simulink model "withaudioip"  (R2016a)
settings: Solver=ode45  StartTime=0.0  StopTime=inf  RelTol=1e-3
libraries: audiosources x1, dspadpt3 x1, dspsnks4 x1
settings Model: Creator=richanetto  LastModifiedBy=richanetto
settings SolverCC: AlgebraicLoopSolver=LineSearch
settings DataIOCC: LimitDataPoints=on
settings DebuggingCC: AlgebraicLoopMsg=none
settings HardwareCC: ProdWordSize=32  ProdHWDeviceType=Specified
settings ModelReferenceCC: PropagateSignalLabelsOutOfModel=off
settings GRTTargetCC: GeneratePreprocessorConditionals=Use local settings

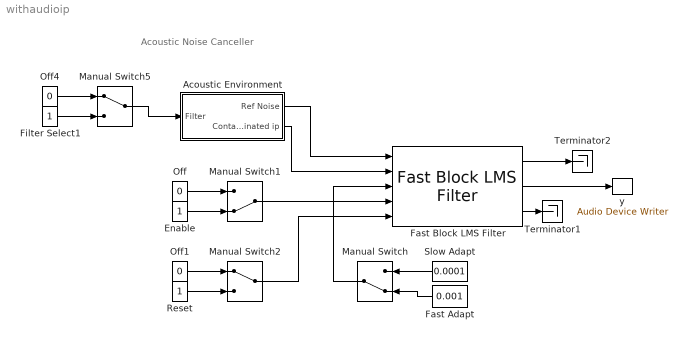
== system withaudioip ==
  note: Acoustic Noise Canceller
  Acoustic Environment : Subsystem
  Enable : Constant  OutDataTypeStr=boolean
  Fast Adapt : Constant  Value=0.001  OutDataTypeStr=Inherit: Inherit via back propagation
  Fast Block LMS Filter : dspadpt3/Fast Block LMS Filter  algo=Fast Block LMS  L=48  N=16  stepflag=Input port  mu=0.008  leakage=1.0  addnparflag=on  ic=0  Adapt=on  resetflag=Non-zero sample  weights=on
  Filter Select1 : Constant  OutDataTypeStr=boolean
  Manual Switch : ManualSwitch  CurrentSetting=0
  Manual Switch1 : ManualSwitch  CurrentSetting=0
  Manual Switch2 : ManualSwitch
  Manual Switch5 : ManualSwitch
  Off : Constant  Value=0  OutDataTypeStr=boolean
  Off1 : Constant  Value=0  OutDataTypeStr=boolean
  Off4 : Constant  Value=0  OutDataTypeStr=boolean
  Reset : Constant  OutDataTypeStr=boolean
  Slow Adapt : Constant  Value=0.0001  OutDataTypeStr=Inherit: Inherit via back propagation
  Terminator1 : Terminator
  Terminator2 : Terminator
  y : dspsnks4/Audio Device Writer  Driver=CoreAudio  Device=Default  InheritSampleRate=on  SampleRate=44100  BitDepth=16-bit integer  BufferSize=4096  NumBuffers=10  DefaultOutputChannelMapping=on  OutputChannelMapping=1:2  OutputNumUnderrunSamples=off  DriverIdx=5  DeviceWarnFlag=''
  wires:
  Slow Adapt/1 -> Manual Switch/1
  Fast Adapt/1 -> Manual Switch/2
  Manual Switch/1 -> Fast Block LMS Filter/3
  Fast Block LMS Filter/3 -> Terminator1/1
  Off/1 -> Manual Switch1/1
  Enable/1 -> Manual Switch1/2
  Off1/1 -> Manual Switch2/1
  Reset/1 -> Manual Switch2/2
  Manual Switch2/1 -> Fast Block LMS Filter/5
  Manual Switch1/1 -> Fast Block LMS Filter/4
  Off4/1 -> Manual Switch5/1
  Filter Select1/1 -> Manual Switch5/2
  Manual Switch5/1 -> Acoustic Environment/1(Filter)
  Acoustic Environment/1(Ref Noise) -> Fast Block LMS Filter/1
  Acoustic Environment/2(Contaminated ip) -> Fast Block LMS Filter/2
  Fast Block LMS Filter/2 -> y/1
  Fast Block LMS Filter/1 -> Terminator2/1

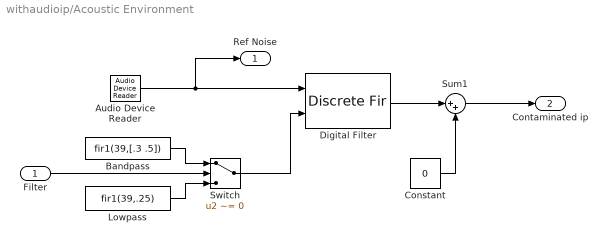
== system withaudioip/Acoustic Environment ==
  Filter : Inport
  Audio Device Reader : audiosources/Audio Device Reader  Driver=CoreAudio  Device=Built-in Microph  SampleRate=44100  NumChannels=1  SamplesPerFrame=1024  BitDepth=16-bit integer  NumBuffers=10  DefaultInputChannelMapping=on  InputChannelMapping=1:2  OutputNumOverrunSamples=off  OutputDataType=double  DriverIdx=5  DeviceWarnFlag=''
  Bandpass : Constant  Value=fir1(39,[.3 .5])  OutDataTypeStr=Inherit: Inherit via back propagation
  Constant : Constant  Value=0
  Digital Filter : DiscreteFir  CoefSource=Input port  Coefficients=[1 2]  InputProcessing=Columns as channels (frame based)  AccumDataTypeStr=Inherit: Same as product output  OutDataTypeStr=Inherit: Same as input
      settings: InputPortMap=u0,u1
  Lowpass : Constant  Value=fir1(39,.25)  OutDataTypeStr=Inherit: Inherit via back propagation
  Sum1 : Sum  Inputs=|++  SaturateOnIntegerOverflow=on  InputSameDT=on  OutDataTypeStr=Inherit: Same as first input
  Switch : Switch  Criteria=u2 ~= 0  SaturateOnIntegerOverflow=on
  Ref Noise : Outport
  Contaminated ip : Outport  Port=2
  wires:
  Constant/1 -> Sum1/2
  Filter/1 -> Switch/2
  Digital Filter/1 -> Sum1/1
  Audio Device Reader/1 -> Ref Noise/1, Digital Filter/1
  Switch/1 -> Digital Filter/2
  Bandpass/1 -> Switch/1
  Lowpass/1 -> Switch/3
  Sum1/1 -> Contaminated ip/1
